simulink model "Fusion_Frame_Model_Architecture"  (R2018a)
settings: Solver=FixedStepAuto  StartTime=0.0  StopTime=SimulationTime  FixedStep=SamplingTime  RelTol=1e-3
undefined symbols (not defined in the file or in its folder): ACTIVATE_CAM, ACTIVATE_RAD, CAM1_detTimeStamp, CAM1_MeasNoise, CAM1_objClassID, CAM1_PX, CAM1_PY, CAM1_VX, CAM1_VY, CAM2_detTimeStamp, CAM2_MeasNoise, CAM2_objClassID, CAM2_PX, CAM2_PY, CAM2_VX, CAM2_VY, CAM3_detTimeStamp, CAM3_MeasNoise, CAM3_objClassID, CAM3_PX, CAM3_PY, CAM3_VX, CAM3_VY, CAM4_detTimeStamp, CAM4_MeasNoise, CAM4_objClassID, CAM4_PX, CAM4_PY, CAM4_VX, CAM4_VY, CAM5_detTimeStamp, CAM5_MeasNoise, CAM5_objClassID, CAM5_PX, CAM5_PY, CAM5_VX, CAM5_VY, CAM6_detTimeStamp, CAM6_MeasNoise, CAM6_objClassID, CAM6_PX, CAM6_PY, CAM6_VX, CAM6_VY, CAM7_detTimeStamp, CAM7_MeasNoise, CAM7_objClassID, CAM7_PX, CAM7_PY, CAM7_VX, CAM7_VY, CAM8_detTimeStamp, CAM8_MeasNoise, CAM8_objClassID, CAM8_PX, CAM8_PY, CAM8_VX, CAM8_VY, CAM_nMeas, CAM_TYPE ... (+181)
libraries: simulink_extras x4
(part 3 of 11)

== system Fusion_Frame_Model_Architecture/SENSOR_MEASUREMENTS/RADAR_CAMERA_EGO_SENSOR_INTERFACE/CameraSensors/Camera7 ==
  timeIdx : Inport
  nObjCamera : Inport  Port=2
  SensorMeas : Inport  Port=3
  ExtractMeasParam1 : Subsystem
  For Iterator : ForIterator  ResetStates=reset  IterationSource=external  IterationVariableDataType=int16
  IsValid2 : Subsystem
  Selector : Selector  InputPortWidth=nCameras  IndexOptions=Starting index (dialog)  Indices=7  OutputSizes=1
  Subsystem1 : Subsystem
  C7 : Outport
  wires:
  ExtractMeasParam1/1(PX) -> IsValid2/2(px), [px]
  ExtractMeasParam1/7(measCaptureTime) -> Subsystem1/9(TIME_STAMP)
  IsValid2/1(ID) -> Subsystem1/6(id)
  [vy] -> Subsystem1/5(vy)  "vy"
  ExtractMeasParam1/6(NOISE_COV) -> Subsystem1/8(NOISE_COV)
  [vx] -> Subsystem1/4(vx)  "vx"
  SensorMeas/1 -> Subsystem1/1(SensorData)
  nObjCamera/1 -> Selector/1
  [py] -> Subsystem1/3(py)  "py"
  For Iterator/1 -> [index]
  [index] -> Subsystem1/10(iter), IsValid2/1(idx), ExtractMeasParam1/1(idx)
  ExtractMeasParam1/4(VY) -> IsValid2/5(vy), [vy]
  [px] -> Subsystem1/2(px)  "px"
  Selector/1 -> For Iterator/1
  ExtractMeasParam1/2(PY) -> IsValid2/3(py), [py]
  Subsystem1/1(C7) -> C7/1
  ExtractMeasParam1/5(OBJ_TYPE) -> Subsystem1/7(OBJ_TYPE)
  timeIdx/1 -> ExtractMeasParam1/2(time)
  ExtractMeasParam1/3(VX) -> IsValid2/4(vx), [vx]

== system Fusion_Frame_Model_Architecture/SENSOR_MEASUREMENTS/RADAR_CAMERA_EGO_SENSOR_INTERFACE/CameraSensors/Camera8 ==
  timeIdx : Inport
  nObjCamera : Inport  Port=2
  SensorMeas : Inport  Port=3
  ExtractMeasParam1 : Subsystem
  For Iterator : ForIterator  ResetStates=reset  IterationSource=external  IterationVariableDataType=int16
  IsValid2 : Subsystem
  Selector : Selector  InputPortWidth=nCameras  IndexOptions=Starting index (dialog)  Indices=8  OutputSizes=1
  Subsystem1 : Subsystem
  C8 : Outport
  wires:
  ExtractMeasParam1/1(PX) -> IsValid2/2(px), [px]
  ExtractMeasParam1/7(measCaptureTime) -> Subsystem1/9(TIME_STAMP)
  IsValid2/1(ID) -> Subsystem1/6(id)
  [vy] -> Subsystem1/5(vy)  "vy"
  ExtractMeasParam1/6(NOISE_COV) -> Subsystem1/8(NOISE_COV)
  [vx] -> Subsystem1/4(vx)  "vx"
  SensorMeas/1 -> Subsystem1/1(SensorData)
  nObjCamera/1 -> Selector/1
  [py] -> Subsystem1/3(py)  "py"
  For Iterator/1 -> [index]
  [index] -> Subsystem1/10(iter), IsValid2/1(idx), ExtractMeasParam1/1(idx)
  ExtractMeasParam1/4(VY) -> IsValid2/5(vy), [vy]
  [px] -> Subsystem1/2(px)  "px"
  Selector/1 -> For Iterator/1
  ExtractMeasParam1/2(PY) -> IsValid2/3(py), [py]
  Subsystem1/1(C8) -> C8/1
  ExtractMeasParam1/5(OBJ_TYPE) -> Subsystem1/7(OBJ_TYPE)
  timeIdx/1 -> ExtractMeasParam1/2(time)
  ExtractMeasParam1/3(VX) -> IsValid2/4(vx), [vx]

== system Fusion_Frame_Model_Architecture/SENSOR_MEASUREMENTS/RADAR_CAMERA_EGO_SENSOR_INTERFACE/EgoSensors/ExtractMeasParam ==
  timeIdx : Inport
  Constant : Constant  Value=EGO_PX
  Constant1 : Constant  Value=EGO_PY
  Constant2 : Constant  Value=EGO_VX
  Constant3 : Constant  Value=EGO_VY
  Constant4 : Constant  Value=EGO_YAW
  Constant5 : Constant  Value=EGO_YAWRATE
  Constant6 : Constant  Value=EGO_TimeStamp
  Constant7 : Constant  Value=EGO_IgnitionStatus
  EGO_PX : Selector  NumberOfDimensions=2  InputPortWidth=portSize  IndexOptions=Select all,Index vector (port)  Indices=[1 3],1  OutputSizes=1,1
  EGO_PY : Selector  NumberOfDimensions=2  InputPortWidth=portSize  IndexOptions=Select all,Index vector (port)  Indices=[1 3],1  OutputSizes=1,1
  EGO_VX : Selector  NumberOfDimensions=2  InputPortWidth=portSize  IndexOptions=Select all,Index vector (port)  Indices=[1 3],1  OutputSizes=1,1
  EGO_VY : Selector  NumberOfDimensions=2  InputPortWidth=portSize  IndexOptions=Select all,Index vector (port)  Indices=[1 3],1  OutputSizes=1,1
  EGO_YAW : Selector  NumberOfDimensions=2  InputPortWidth=portSize  IndexOptions=Select all,Index vector (port)  Indices=[1 3],1  OutputSizes=1,1
  EGO_YAWRATE : Selector  NumberOfDimensions=2  InputPortWidth=portSize  IndexOptions=Select all,Index vector (port)  Indices=[1 3],1  OutputSizes=1,1
  TIME_STAMP : Selector  NumberOfDimensions=2  InputPortWidth=portSize  IndexOptions=Select all,Index vector (port)  Indices=[1 3],1  OutputSizes=1,1
  TIME_STAMP1 : Selector  NumberOfDimensions=2  InputPortWidth=portSize  IndexOptions=Select all,Index vector (port)  Indices=[1 3],1  OutputSizes=1,1
  EgoTimeStamp : Outport
  EgoPx : Outport  Port=2
  EgoPy : Outport  Port=3
  EgoVx : Outport  Port=4
  EgoVy : Outport  Port=5
  EgoYaw : Outport  Port=6
  EgoYawRate : Outport  Port=7
  EgoIgnitionStatus : Outport  Port=8
  wires:
  Constant3/1 -> EGO_VY/1
  Constant2/1 -> EGO_VX/1
  Constant/1 -> EGO_PX/1
  Constant1/1 -> EGO_PY/1
  EGO_VX/1 -> EgoVx/1
  EGO_PX/1 -> EgoPx/1
  timeIdx/1 -> EGO_PX/2, EGO_PY/2, EGO_VX/2, EGO_VY/2, EGO_YAW/2, EGO_YAWRATE/2, TIME_STAMP1/2, TIME_STAMP/2
  Constant4/1 -> EGO_YAW/1
  EGO_YAW/1 -> EgoYaw/1
  Constant6/1 -> TIME_STAMP/1
  TIME_STAMP/1 -> EgoTimeStamp/1
  EGO_YAWRATE/1 -> EgoYawRate/1
  Constant5/1 -> EGO_YAWRATE/1
  EGO_PY/1 -> EgoPy/1
  EGO_VY/1 -> EgoVy/1
  Constant7/1 -> TIME_STAMP1/1
  TIME_STAMP1/1 -> EgoIgnitionStatus/1

== system Fusion_Frame_Model_Architecture/SENSOR_MEASUREMENTS/RADAR_CAMERA_EGO_SENSOR_INTERFACE/RadarSensors/Radar1 ==
  timeIdx : Inport
  nObjRadar : Inport  Port=2
  SensorMeas : Inport  Port=3
  CHECK_IF_DATA_VALID : Subsystem
  GET_DATA : Subsystem
  LOOP_OVER_RADARS : ForIterator  ResetStates=reset  IterationSource=external  IterationVariableDataType=int16
  SET_DATA : Subsystem
  Selector : Selector  InputPortWidth=nRadars  IndexOptions=Starting index (dialog)  Indices=1  OutputSizes=1
  R1 : Outport
  wires:
  nObjRadar/1 -> Selector/1
  LOOP_OVER_RADARS/1 -> [index]
  [index] -> CHECK_IF_DATA_VALID/1(idx), GET_DATA/1(idx), SET_DATA/10(iter)
  timeIdx/1 -> GET_DATA/2(time)
  GET_DATA/1(PX) -> CHECK_IF_DATA_VALID/2(px), [px]
  GET_DATA/2(PY) -> CHECK_IF_DATA_VALID/3(py), [py]
  GET_DATA/3(VX) -> CHECK_IF_DATA_VALID/4(vx), [vx]
  GET_DATA/4(VY) -> CHECK_IF_DATA_VALID/5(vy), [vy]
  SensorMeas/1 -> SET_DATA/1(SensorData)
  [px] -> SET_DATA/2(px)  "px"
  [py] -> SET_DATA/3(py)  "py"
  [vx] -> SET_DATA/4(vx)  "vx"
  [vy] -> SET_DATA/5(vy)  "vy"
  SET_DATA/1(R1) -> R1/1
  CHECK_IF_DATA_VALID/1(ID) -> SET_DATA/6(id)
  Selector/1 -> LOOP_OVER_RADARS/1
  GET_DATA/5(SNR) -> SET_DATA/7(SNR)
  GET_DATA/6(NOISE_COV) -> SET_DATA/8(NOISE_COV)
  GET_DATA/7(measCaptureTime) -> SET_DATA/9(TIME_STAMP)

== system Fusion_Frame_Model_Architecture/SENSOR_MEASUREMENTS/RADAR_CAMERA_EGO_SENSOR_INTERFACE/RadarSensors/Radar2 ==
  timeIdx : Inport
  nObjRadar : Inport  Port=2
  SensorMeas : Inport  Port=3
  ExtractMeasParam : Subsystem
  For Iterator : ForIterator  ResetStates=reset  IterationSource=external  IterationVariableDataType=int16
  IsValid1 : Subsystem
  Selector : Selector  InputPortWidth=nRadars  IndexOptions=Starting index (dialog)  Indices=2  OutputSizes=1
  Subsystem : Subsystem
  R2 : Outport
  wires:
  [vx] -> Subsystem/4(vx)  "vx"
  Subsystem/1(R2) -> R2/1
  ExtractMeasParam/1(PX) -> IsValid1/2(px), [px]
  IsValid1/1(ID) -> Subsystem/6(id)
  [py] -> Subsystem/3(py)  "py"
  ExtractMeasParam/3(VX) -> IsValid1/4(vx), [vx]
  ExtractMeasParam/6(NOISE_COV) -> Subsystem/8(NOISE_COV)
  ExtractMeasParam/4(VY) -> IsValid1/5(vy), [vy]
  [px] -> Subsystem/2(px)  "px"
  nObjRadar/1 -> Selector/1
  SensorMeas/1 -> Subsystem/1(SensorData)
  timeIdx/1 -> ExtractMeasParam/2(time)
  [index] -> IsValid1/1(idx), ExtractMeasParam/1(idx), Subsystem/10(iter)
  [vy] -> Subsystem/5(vy)  "vy"
  ExtractMeasParam/2(PY) -> IsValid1/3(py), [py]
  For Iterator/1 -> [index]
  ExtractMeasParam/5(SNR) -> Subsystem/7(SNR)
  ExtractMeasParam/7(measCaptureTime) -> Subsystem/9(TIME_STAMP)
  Selector/1 -> For Iterator/1

== system Fusion_Frame_Model_Architecture/SENSOR_MEASUREMENTS/RADAR_CAMERA_EGO_SENSOR_INTERFACE/RadarSensors/Radar3 ==
  timeIdx : Inport
  nObjRadar : Inport  Port=2
  SensorMeas : Inport  Port=3
  ExtractMeasParam : Subsystem
  For Iterator : ForIterator  ResetStates=reset  IterationSource=external  IterationVariableDataType=int16
  IsValid1 : Subsystem
  Selector : Selector  InputPortWidth=nRadars  IndexOptions=Starting index (dialog)  Indices=3  OutputSizes=1
  Subsystem : Subsystem
  R3 : Outport
  wires:
  [vx] -> Subsystem/4(vx)  "vx"
  Subsystem/1(R3) -> R3/1
  ExtractMeasParam/1(PX) -> IsValid1/2(px), [px]
  IsValid1/1(ID) -> Subsystem/6(id)
  [py] -> Subsystem/3(py)  "py"
  ExtractMeasParam/3(VX) -> IsValid1/4(vx), [vx]
  ExtractMeasParam/6(NOISE_COV) -> Subsystem/8(NOISE_COV)
  ExtractMeasParam/4(VY) -> IsValid1/5(vy), [vy]
  [px] -> Subsystem/2(px)  "px"
  nObjRadar/1 -> Selector/1
  SensorMeas/1 -> Subsystem/1(SensorData)
  timeIdx/1 -> ExtractMeasParam/2(time)
  [index] -> IsValid1/1(idx), ExtractMeasParam/1(idx), Subsystem/10(iter)
  [vy] -> Subsystem/5(vy)  "vy"
  ExtractMeasParam/2(PY) -> IsValid1/3(py), [py]
  For Iterator/1 -> [index]
  ExtractMeasParam/5(SNR) -> Subsystem/7(SNR)
  ExtractMeasParam/7(measCaptureTime) -> Subsystem/9(TIME_STAMP)
  Selector/1 -> For Iterator/1

== system Fusion_Frame_Model_Architecture/SENSOR_MEASUREMENTS/RADAR_CAMERA_EGO_SENSOR_INTERFACE/RadarSensors/Radar4 ==
  timeIdx : Inport
  nObjRadar : Inport  Port=2
  SensorMeas : Inport  Port=3
  ExtractMeasParam : Subsystem
  For Iterator : ForIterator  ResetStates=reset  IterationSource=external  IterationVariableDataType=int16
  IsValid1 : Subsystem
  Selector : Selector  InputPortWidth=nRadars  IndexOptions=Starting index (dialog)  Indices=4  OutputSizes=1
  Subsystem : Subsystem
  R4 : Outport
  wires:
  ExtractMeasParam/2(PY) -> IsValid1/3(py), [py]
  [vy] -> Subsystem/5(vy)  "vy"
  [index] -> IsValid1/1(idx), ExtractMeasParam/1(idx), Subsystem/10(iter)
  SensorMeas/1 -> Subsystem/1(SensorData)
  ExtractMeasParam/6(NOISE_COV) -> Subsystem/8(NOISE_COV)
  ExtractMeasParam/4(VY) -> IsValid1/5(vy), [vy]
  ExtractMeasParam/3(VX) -> IsValid1/4(vx), [vx]
  timeIdx/1 -> ExtractMeasParam/2(time)
  IsValid1/1(ID) -> Subsystem/6(id)
  ExtractMeasParam/1(PX) -> IsValid1/2(px), [px]
  [vx] -> Subsystem/4(vx)  "vx"
  Selector/1 -> For Iterator/1
  nObjRadar/1 -> Selector/1
  Subsystem/1(R4) -> R4/1
  ExtractMeasParam/7(measCaptureTime) -> Subsystem/9(TIME_STAMP)
  [px] -> Subsystem/2(px)  "px"
  ExtractMeasParam/5(SNR) -> Subsystem/7(SNR)
  [py] -> Subsystem/3(py)  "py"
  For Iterator/1 -> [index]

== system Fusion_Frame_Model_Architecture/SENSOR_MEASUREMENTS/RADAR_CAMERA_EGO_SENSOR_INTERFACE/RadarSensors/Radar5 ==
  timeIdx : Inport
  nObjRadar : Inport  Port=2
  SensorMeas : Inport  Port=3
  ExtractMeasParam : Subsystem
  For Iterator : ForIterator  ResetStates=reset  IterationSource=external  IterationVariableDataType=int16
  IsValid1 : Subsystem
  Selector : Selector  InputPortWidth=nRadars  IndexOptions=Starting index (dialog)  Indices=5  OutputSizes=1
  Subsystem : Subsystem
  R5 : Outport
  wires:
  ExtractMeasParam/2(PY) -> IsValid1/3(py), [py]
  [vy] -> Subsystem/5(vy)  "vy"
  [index] -> IsValid1/1(idx), ExtractMeasParam/1(idx), Subsystem/10(iter)
  SensorMeas/1 -> Subsystem/1(SensorData)
  ExtractMeasParam/6(NOISE_COV) -> Subsystem/8(NOISE_COV)
  ExtractMeasParam/4(VY) -> IsValid1/5(vy), [vy]
  ExtractMeasParam/3(VX) -> IsValid1/4(vx), [vx]
  timeIdx/1 -> ExtractMeasParam/2(time)
  IsValid1/1(ID) -> Subsystem/6(id)
  ExtractMeasParam/1(PX) -> IsValid1/2(px), [px]
  [vx] -> Subsystem/4(vx)  "vx"
  Selector/1 -> For Iterator/1
  nObjRadar/1 -> Selector/1
  Subsystem/1(R5) -> R5/1
  ExtractMeasParam/7(measCaptureTime) -> Subsystem/9(TIME_STAMP)
  [px] -> Subsystem/2(px)  "px"
  ExtractMeasParam/5(SNR) -> Subsystem/7(SNR)
  [py] -> Subsystem/3(py)  "py"
  For Iterator/1 -> [index]

== system Fusion_Frame_Model_Architecture/SENSOR_MEASUREMENTS/RADAR_CAMERA_EGO_SENSOR_INTERFACE/RadarSensors/Radar6 ==
  timeIdx : Inport
  nObjRadar : Inport  Port=2
  SensorMeas : Inport  Port=3
  ExtractMeasParam : Subsystem
  For Iterator : ForIterator  ResetStates=reset  IterationSource=external  IterationVariableDataType=int16
  IsValid1 : Subsystem
  Selector : Selector  InputPortWidth=nRadars  IndexOptions=Starting index (dialog)  Indices=6  OutputSizes=1
  Subsystem : Subsystem
  R6 : Outport
  wires:
  ExtractMeasParam/2(PY) -> IsValid1/3(py), [py]
  [vy] -> Subsystem/5(vy)  "vy"
  [index] -> IsValid1/1(idx), ExtractMeasParam/1(idx), Subsystem/10(iter)
  SensorMeas/1 -> Subsystem/1(SensorData)
  ExtractMeasParam/6(NOISE_COV) -> Subsystem/8(NOISE_COV)
  ExtractMeasParam/4(VY) -> IsValid1/5(vy), [vy]
  ExtractMeasParam/3(VX) -> IsValid1/4(vx), [vx]
  timeIdx/1 -> ExtractMeasParam/2(time)
  IsValid1/1(ID) -> Subsystem/6(id)
  ExtractMeasParam/1(PX) -> IsValid1/2(px), [px]
  [vx] -> Subsystem/4(vx)  "vx"
  Selector/1 -> For Iterator/1
  nObjRadar/1 -> Selector/1
  Subsystem/1(R6) -> R6/1
  ExtractMeasParam/7(measCaptureTime) -> Subsystem/9(TIME_STAMP)
  [px] -> Subsystem/2(px)  "px"
  ExtractMeasParam/5(SNR) -> Subsystem/7(SNR)
  [py] -> Subsystem/3(py)  "py"
  For Iterator/1 -> [index]

== system Fusion_Frame_Model_Architecture/SENSOR_MEASUREMENTS/RADAR_CAMERA_EGO_SENSOR_INTERFACE/RoadSensors/Camera1 ==
  timeIdx : Inport
  nLines : Inport  Port=2
  CameraLineCoeff : Inport  Port=3
  CHECK_IF_DATA_IS_VALID : Subsystem
  GET_DATA : Subsystem
  LOOP_OVER_CAMERAS : ForIterator  ResetStates=reset  IterationSource=external  IterationVariableDataType=int16
  SET_DATA : Subsystem
  Selector : Selector  InputPortWidth=nCameras  IndexOptions=Index vector (dialog)  Indices=1  OutputSizes=1
  C1 : Outport
  wires:
  nLines/1 -> Selector/1
  LOOP_OVER_CAMERAS/1 -> [index]
  GET_DATA/5(lateralOffset) -> SET_DATA/7(lateralOffset)
  [curv] -> SET_DATA/2(curv)
  GET_DATA/9(measCaptureTime) -> SET_DATA/11(TIME_STAMP)
  SET_DATA/1(C1) -> C1/1
  [curvLen] -> SET_DATA/4(curvLen)
  GET_DATA/1(curvature) -> CHECK_IF_DATA_IS_VALID/2(curvature), [curv]
  Selector/1 -> LOOP_OVER_CAMERAS/1
  GET_DATA/3(curvLength) -> CHECK_IF_DATA_IS_VALID/4(curvLength), [curvLen]
  timeIdx/1 -> GET_DATA/2(time)
  CHECK_IF_DATA_IS_VALID/1(validID) -> SET_DATA/6(ValidID)
  CameraLineCoeff/1 -> SET_DATA/1(CameraLineCoeff)
  GET_DATA/6(xmin) -> SET_DATA/8(xmin)
  [alpha] -> SET_DATA/5(alpha)
  [curvRate] -> SET_DATA/3(curvRate)
  GET_DATA/4(headingAngle) -> CHECK_IF_DATA_IS_VALID/5(HeadingAngle), [alpha]
  GET_DATA/2(curvRate) -> CHECK_IF_DATA_IS_VALID/3(curvatureRate), [curvRate]
  [index] -> CHECK_IF_DATA_IS_VALID/1(LineID), SET_DATA/12(iter), GET_DATA/1(idx)
  GET_DATA/7(xmax) -> SET_DATA/9(xmax)
  GET_DATA/8(lineMarkWidth) -> SET_DATA/10(lineWidth)

== system Fusion_Frame_Model_Architecture/SENSOR_MEASUREMENTS/RADAR_CAMERA_EGO_SENSOR_INTERFACE/RoadSensors/Camera2 ==
  timeIdx : Inport
  nLines : Inport  Port=2
  CameraLineCoeff : Inport  Port=3
  ExtractMeasParam1 : Subsystem
  For Iterator : ForIterator  ResetStates=reset  IterationSource=external  IterationVariableDataType=int16
  IsValid2 : Subsystem
  Selector : Selector  InputPortWidth=nCameras  IndexOptions=Index vector (dialog)  Indices=2  OutputSizes=1
  Subsystem1 : Subsystem
  C1 : Outport
  wires:
  ExtractMeasParam1/7(xmax) -> Subsystem1/9(xmax)
  ExtractMeasParam1/8(lineMarkWidth) -> Subsystem1/10(lineWidth)
  [index] -> IsValid2/1(LineID), Subsystem1/12(iter), ExtractMeasParam1/1(idx)
  timeIdx/1 -> ExtractMeasParam1/2(time)
  ExtractMeasParam1/2(curvRate) -> IsValid2/3(curvatureRate), [curvRate]
  [curvRate] -> Subsystem1/3(curvRate)
  [curv] -> Subsystem1/2(curv)
  ExtractMeasParam1/3(curvLength) -> IsValid2/4(curvLength), [curvLen]
  ExtractMeasParam1/1(curvature) -> IsValid2/2(curvature), [curv]
  Subsystem1/1(C1) -> C1/1
  [curvLen] -> Subsystem1/4(curvLen)
  For Iterator/1 -> [index]
  ExtractMeasParam1/4(headingAngle) -> IsValid2/5(HeadingAngle), [alpha]
  ExtractMeasParam1/5(lateralOffset) -> Subsystem1/7(lateralOffset)
  Selector/1 -> For Iterator/1
  IsValid2/1(validID) -> Subsystem1/6(ValidID)
  ExtractMeasParam1/6(xmin) -> Subsystem1/8(xmin)
  CameraLineCoeff/1 -> Subsystem1/1(CameraLineCoeff)
  nLines/1 -> Selector/1
  ExtractMeasParam1/9(measCaptureTime) -> Subsystem1/11(TIME_STAMP)
  [alpha] -> Subsystem1/5(alpha)

== system Fusion_Frame_Model_Architecture/SENSOR_MEASUREMENTS/RADAR_CAMERA_EGO_SENSOR_INTERFACE/RoadSensors/Camera3 ==
  timeIdx : Inport
  nLines : Inport  Port=2
  CameraLineCoeff : Inport  Port=3
  ExtractMeasParam1 : Subsystem
  For Iterator : ForIterator  ResetStates=reset  IterationSource=external  IterationVariableDataType=int16
  IsValid2 : Subsystem
  Selector : Selector  InputPortWidth=nCameras  IndexOptions=Index vector (dialog)  Indices=3  OutputSizes=1
  Subsystem1 : Subsystem
  C1 : Outport
  wires:
  ExtractMeasParam1/7(xmax) -> Subsystem1/9(xmax)
  ExtractMeasParam1/8(lineMarkWidth) -> Subsystem1/10(lineWidth)
  [index] -> IsValid2/1(LineID), Subsystem1/12(iter), ExtractMeasParam1/1(idx)
  timeIdx/1 -> ExtractMeasParam1/2(time)
  ExtractMeasParam1/2(curvRate) -> IsValid2/3(curvatureRate), [curvRate]
  [curvRate] -> Subsystem1/3(curvRate)
  [curv] -> Subsystem1/2(curv)
  ExtractMeasParam1/3(curvLength) -> IsValid2/4(curvLength), [curvLen]
  ExtractMeasParam1/1(curvature) -> IsValid2/2(curvature), [curv]
  Subsystem1/1(C1) -> C1/1
  [curvLen] -> Subsystem1/4(curvLen)
  For Iterator/1 -> [index]
  ExtractMeasParam1/4(headingAngle) -> IsValid2/5(HeadingAngle), [alpha]
  ExtractMeasParam1/5(lateralOffset) -> Subsystem1/7(lateralOffset)
  Selector/1 -> For Iterator/1
  IsValid2/1(validID) -> Subsystem1/6(ValidID)
  ExtractMeasParam1/6(xmin) -> Subsystem1/8(xmin)
  CameraLineCoeff/1 -> Subsystem1/1(CameraLineCoeff)
  nLines/1 -> Selector/1
  ExtractMeasParam1/9(measCaptureTime) -> Subsystem1/11(TIME_STAMP)
  [alpha] -> Subsystem1/5(alpha)

== system Fusion_Frame_Model_Architecture/SENSOR_MEASUREMENTS/RADAR_CAMERA_EGO_SENSOR_INTERFACE/RoadSensors/Camera4 ==
  timeIdx : Inport
  nLines : Inport  Port=2
  CameraLineCoeff : Inport  Port=3
  ExtractMeasParam1 : Subsystem
  For Iterator : ForIterator  ResetStates=reset  IterationSource=external  IterationVariableDataType=int16
  IsValid2 : Subsystem
  Selector : Selector  InputPortWidth=nCameras  IndexOptions=Index vector (dialog)  Indices=4  OutputSizes=1
  Subsystem1 : Subsystem
  C1 : Outport
  wires:
  ExtractMeasParam1/7(xmax) -> Subsystem1/9(xmax)
  ExtractMeasParam1/8(lineMarkWidth) -> Subsystem1/10(lineWidth)
  [index] -> IsValid2/1(LineID), Subsystem1/12(iter), ExtractMeasParam1/1(idx)
  timeIdx/1 -> ExtractMeasParam1/2(time)
  ExtractMeasParam1/2(curvRate) -> IsValid2/3(curvatureRate), [curvRate]
  [curvRate] -> Subsystem1/3(curvRate)
  [curv] -> Subsystem1/2(curv)
  ExtractMeasParam1/3(curvLength) -> IsValid2/4(curvLength), [curvLen]
  ExtractMeasParam1/1(curvature) -> IsValid2/2(curvature), [curv]
  Subsystem1/1(C1) -> C1/1
  [curvLen] -> Subsystem1/4(curvLen)
  For Iterator/1 -> [index]
  ExtractMeasParam1/4(headingAngle) -> IsValid2/5(HeadingAngle), [alpha]
  ExtractMeasParam1/5(lateralOffset) -> Subsystem1/7(lateralOffset)
  Selector/1 -> For Iterator/1
  IsValid2/1(validID) -> Subsystem1/6(ValidID)
  ExtractMeasParam1/6(xmin) -> Subsystem1/8(xmin)
  CameraLineCoeff/1 -> Subsystem1/1(CameraLineCoeff)
  nLines/1 -> Selector/1
  ExtractMeasParam1/9(measCaptureTime) -> Subsystem1/11(TIME_STAMP)
  [alpha] -> Subsystem1/5(alpha)

== system Fusion_Frame_Model_Architecture/SENSOR_MEASUREMENTS/RADAR_CAMERA_EGO_SENSOR_INTERFACE/RoadSensors/Camera5 ==
  timeIdx : Inport
  nLines : Inport  Port=2
  CameraLineCoeff : Inport  Port=3
  ExtractMeasParam1 : Subsystem
  For Iterator : ForIterator  ResetStates=reset  IterationSource=external  IterationVariableDataType=int16
  IsValid2 : Subsystem
  Selector : Selector  InputPortWidth=nCameras  IndexOptions=Index vector (dialog)  Indices=5  OutputSizes=1
  Subsystem1 : Subsystem
  C1 : Outport
  wires:
  ExtractMeasParam1/7(xmax) -> Subsystem1/9(xmax)
  ExtractMeasParam1/8(lineMarkWidth) -> Subsystem1/10(lineWidth)
  [index] -> IsValid2/1(LineID), Subsystem1/12(iter), ExtractMeasParam1/1(idx)
  timeIdx/1 -> ExtractMeasParam1/2(time)
  ExtractMeasParam1/2(curvRate) -> IsValid2/3(curvatureRate), [curvRate]
  [curvRate] -> Subsystem1/3(curvRate)
  [curv] -> Subsystem1/2(curv)
  ExtractMeasParam1/3(curvLength) -> IsValid2/4(curvLength), [curvLen]
  ExtractMeasParam1/1(curvature) -> IsValid2/2(curvature), [curv]
  Subsystem1/1(C1) -> C1/1
  [curvLen] -> Subsystem1/4(curvLen)
  For Iterator/1 -> [index]
  ExtractMeasParam1/4(headingAngle) -> IsValid2/5(HeadingAngle), [alpha]
  ExtractMeasParam1/5(lateralOffset) -> Subsystem1/7(lateralOffset)
  Selector/1 -> For Iterator/1
  IsValid2/1(validID) -> Subsystem1/6(ValidID)
  ExtractMeasParam1/6(xmin) -> Subsystem1/8(xmin)
  CameraLineCoeff/1 -> Subsystem1/1(CameraLineCoeff)
  nLines/1 -> Selector/1
  ExtractMeasParam1/9(measCaptureTime) -> Subsystem1/11(TIME_STAMP)
  [alpha] -> Subsystem1/5(alpha)

== system Fusion_Frame_Model_Architecture/SENSOR_MEASUREMENTS/RADAR_CAMERA_EGO_SENSOR_INTERFACE/RoadSensors/Camera6 ==
  timeIdx : Inport
  nLines : Inport  Port=2
  CameraLineCoeff : Inport  Port=3
  ExtractMeasParam1 : Subsystem
  For Iterator : ForIterator  ResetStates=reset  IterationSource=external  IterationVariableDataType=int16
  IsValid2 : Subsystem
  Selector : Selector  InputPortWidth=nCameras  IndexOptions=Index vector (dialog)  Indices=6  OutputSizes=1
  Subsystem1 : Subsystem
  C1 : Outport
  wires:
  ExtractMeasParam1/7(xmax) -> Subsystem1/9(xmax)
  ExtractMeasParam1/8(lineMarkWidth) -> Subsystem1/10(lineWidth)
  [index] -> IsValid2/1(LineID), Subsystem1/12(iter), ExtractMeasParam1/1(idx)
  timeIdx/1 -> ExtractMeasParam1/2(time)
  ExtractMeasParam1/2(curvRate) -> IsValid2/3(curvatureRate), [curvRate]
  [curvRate] -> Subsystem1/3(curvRate)
  [curv] -> Subsystem1/2(curv)
  ExtractMeasParam1/3(curvLength) -> IsValid2/4(curvLength), [curvLen]
  ExtractMeasParam1/1(curvature) -> IsValid2/2(curvature), [curv]
  Subsystem1/1(C1) -> C1/1
  [curvLen] -> Subsystem1/4(curvLen)
  For Iterator/1 -> [index]
  ExtractMeasParam1/4(headingAngle) -> IsValid2/5(HeadingAngle), [alpha]
  ExtractMeasParam1/5(lateralOffset) -> Subsystem1/7(lateralOffset)
  Selector/1 -> For Iterator/1
  IsValid2/1(validID) -> Subsystem1/6(ValidID)
  ExtractMeasParam1/6(xmin) -> Subsystem1/8(xmin)
  CameraLineCoeff/1 -> Subsystem1/1(CameraLineCoeff)
  nLines/1 -> Selector/1
  ExtractMeasParam1/9(measCaptureTime) -> Subsystem1/11(TIME_STAMP)
  [alpha] -> Subsystem1/5(alpha)

== system Fusion_Frame_Model_Architecture/SENSOR_MEASUREMENTS/RADAR_CAMERA_EGO_SENSOR_INTERFACE/RoadSensors/Camera7 ==
  timeIdx : Inport
  nLines : Inport  Port=2
  CameraLineCoeff : Inport  Port=3
  ExtractMeasParam1 : Subsystem
  For Iterator : ForIterator  ResetStates=reset  IterationSource=external  IterationVariableDataType=int16
  IsValid2 : Subsystem
  Selector : Selector  InputPortWidth=nCameras  IndexOptions=Index vector (dialog)  Indices=7  OutputSizes=1
  Subsystem1 : Subsystem
  C1 : Outport
  wires:
  ExtractMeasParam1/7(xmax) -> Subsystem1/9(xmax)
  ExtractMeasParam1/8(lineMarkWidth) -> Subsystem1/10(lineWidth)
  [index] -> IsValid2/1(LineID), Subsystem1/12(iter), ExtractMeasParam1/1(idx)
  timeIdx/1 -> ExtractMeasParam1/2(time)
  ExtractMeasParam1/2(curvRate) -> IsValid2/3(curvatureRate), [curvRate]
  [curvRate] -> Subsystem1/3(curvRate)
  [curv] -> Subsystem1/2(curv)
  ExtractMeasParam1/3(curvLength) -> IsValid2/4(curvLength), [curvLen]
  ExtractMeasParam1/1(curvature) -> IsValid2/2(curvature), [curv]
  Subsystem1/1(C1) -> C1/1
  [curvLen] -> Subsystem1/4(curvLen)
  For Iterator/1 -> [index]
  ExtractMeasParam1/4(headingAngle) -> IsValid2/5(HeadingAngle), [alpha]
  ExtractMeasParam1/5(lateralOffset) -> Subsystem1/7(lateralOffset)
  Selector/1 -> For Iterator/1
  IsValid2/1(validID) -> Subsystem1/6(ValidID)
  ExtractMeasParam1/6(xmin) -> Subsystem1/8(xmin)
  CameraLineCoeff/1 -> Subsystem1/1(CameraLineCoeff)
  nLines/1 -> Selector/1
  ExtractMeasParam1/9(measCaptureTime) -> Subsystem1/11(TIME_STAMP)
  [alpha] -> Subsystem1/5(alpha)

== system Fusion_Frame_Model_Architecture/SENSOR_MEASUREMENTS/RADAR_CAMERA_EGO_SENSOR_INTERFACE/RoadSensors/Camera8 ==
  timeIdx : Inport
  nLines : Inport  Port=2
  CameraLineCoeff : Inport  Port=3
  ExtractMeasParam1 : Subsystem
  For Iterator : ForIterator  ResetStates=reset  IterationSource=external  IterationVariableDataType=int16
  IsValid2 : Subsystem
  Selector : Selector  InputPortWidth=nCameras  IndexOptions=Index vector (dialog)  Indices=8  OutputSizes=1
  Subsystem1 : Subsystem
  C1 : Outport
  wires:
  ExtractMeasParam1/7(xmax) -> Subsystem1/9(xmax)
  ExtractMeasParam1/8(lineMarkWidth) -> Subsystem1/10(lineWidth)
  [index] -> IsValid2/1(LineID), Subsystem1/12(iter), ExtractMeasParam1/1(idx)
  timeIdx/1 -> ExtractMeasParam1/2(time)
  ExtractMeasParam1/2(curvRate) -> IsValid2/3(curvatureRate), [curvRate]
  [curvRate] -> Subsystem1/3(curvRate)
  [curv] -> Subsystem1/2(curv)
  ExtractMeasParam1/3(curvLength) -> IsValid2/4(curvLength), [curvLen]
  ExtractMeasParam1/1(curvature) -> IsValid2/2(curvature), [curv]
  Subsystem1/1(C1) -> C1/1
  [curvLen] -> Subsystem1/4(curvLen)
  For Iterator/1 -> [index]
  ExtractMeasParam1/4(headingAngle) -> IsValid2/5(HeadingAngle), [alpha]
  ExtractMeasParam1/5(lateralOffset) -> Subsystem1/7(lateralOffset)
  Selector/1 -> For Iterator/1
  IsValid2/1(validID) -> Subsystem1/6(ValidID)
  ExtractMeasParam1/6(xmin) -> Subsystem1/8(xmin)
  CameraLineCoeff/1 -> Subsystem1/1(CameraLineCoeff)
  nLines/1 -> Selector/1
  ExtractMeasParam1/9(measCaptureTime) -> Subsystem1/11(TIME_STAMP)
  [alpha] -> Subsystem1/5(alpha)

== system Fusion_Frame_Model_Architecture/SENSOR_FUSION_SYSTEM/OBJECT_TRACKER_SENSOR_FUSION/CAMERA_HOMOGENEOUS_FUSION/GATING/FIND_UNASSOCIATED_CLUSTERS ==
  GatedMeasFlagArray : Inport
  Clusters : Inport  Port=2
  measCLUSTERS : Inport  Port=3
  Terminator : Terminator
  Terminator1 : Terminator
  UngatedCLUSTERS : Outport
  wires:
  measCLUSTERS/1 -> UngatedCLUSTERS/1
  GatedMeasFlagArray/1 -> Terminator/1
  Clusters/1 -> Terminator1/1

== system Fusion_Frame_Model_Architecture/SENSOR_FUSION_SYSTEM/OBJECT_TRACKER_SENSOR_FUSION/CAMERA_HOMOGENEOUS_FUSION/GATING/GET_DATA ==
  TRACKS : Inport
  Bus Selector : BusSelector  OutputSignals=nValidTracks,TrackParam
  nTracksPred : Outport
  TrackParam : Outport  Port=2
  wires:
  TRACKS/1 -> Bus Selector/1
  Bus Selector/1 -> nTracksPred/1  "<nValidTracks>"
  Bus Selector/2 -> TrackParam/1  "<TrackParam>"

== system Fusion_Frame_Model_Architecture/SENSOR_FUSION_SYSTEM/OBJECT_TRACKER_SENSOR_FUSION/CAMERA_HOMOGENEOUS_FUSION/GATING/MEASUREMENT_TO_TRACK_GATING_AND_LOGLIKELIHOOD_COMPUTATION ==
  nTracks : Inport
  TrackParamPred : Inport  Port=2
  SnsrParam : Inport  Port=3
  Meas : Inport  Port=4
  For Iterator : ForIterator  ResetStates=reset  IterationSource=external
  GATE_MEASUREMENTS_AND_COMPUTE_LIKELIHOOD : Subsystem
  GET_DATA : Subsystem
  Terminator : Terminator
  Unit Delay : UnitDelay  InitialCondition=boolean(zeros(100, 1200))  SampleTime=-1
  Unit Delay1 : UnitDelay  InitialCondition=single(zeros(100, 1200))  SampleTime=-1
  nMeas : Outport
  GatedMeasFlagArray : Outport  Port=2
  GatedMeasLogLikelihood : Outport  Port=3
  wires:
  GATE_MEASUREMENTS_AND_COMPUTE_LIKELIHOOD/1(GatedMeasFlagArray) -> GatedMeasFlagArray/1, Unit Delay/1
  nTracks/1 -> For Iterator/1
  TrackParamPred/1 -> GET_DATA/2(TrackParamPred)
  GATE_MEASUREMENTS_AND_COMPUTE_LIKELIHOOD/2(LogLikelihoodArray) -> Unit Delay1/1, GatedMeasLogLikelihood/1
  GET_DATA/2(StateVector) -> GATE_MEASUREMENTS_AND_COMPUTE_LIKELIHOOD/4(TrackStateVector)
  GET_DATA/3(StateErrCov) -> GATE_MEASUREMENTS_AND_COMPUTE_LIKELIHOOD/5(TrackErrCov)
  For Iterator/1 -> GATE_MEASUREMENTS_AND_COMPUTE_LIKELIHOOD/6(TrackIdx), GET_DATA/3(TrackIdx)
  Meas/1 -> GATE_MEASUREMENTS_AND_COMPUTE_LIKELIHOOD/2(Meas), GET_DATA/1(Meas)
  GET_DATA/1(nMeas) -> [nMeas], GATE_MEASUREMENTS_AND_COMPUTE_LIKELIHOOD/3(nMeas)
  Unit Delay1/1 -> GATE_MEASUREMENTS_AND_COMPUTE_LIKELIHOOD/7(LogLikelihoodArrayIn)
  Unit Delay/1 -> GATE_MEASUREMENTS_AND_COMPUTE_LIKELIHOOD/1(GatedMeasFlagArrayIn)
  [nMeas] -> nMeas/1
  SnsrParam/1 -> Terminator/1

== system Fusion_Frame_Model_Architecture/SENSOR_FUSION_SYSTEM/OBJECT_TRACKER_SENSOR_FUSION/CAMERA_HOMOGENEOUS_FUSION/GATING/RESOLVE_GATING_AMBIGUITY ==
  nTracks : Inport
  nMeas : Inport  Port=2
  GatedMeasFlagArrayIn : Inport  Port=3
  GatedMeasLogLikelihoodIn : Inport  Port=4
  Terminator : Terminator
  Terminator1 : Terminator
  GatedMeasFlagArray : Outport
  GatedMeasLogLikelihood : Outport  Port=2
  wires:
  nTracks/1 -> Terminator/1
  GatedMeasLogLikelihoodIn/1 -> GatedMeasLogLikelihood/1
  GatedMeasFlagArrayIn/1 -> GatedMeasFlagArray/1
  nMeas/1 -> Terminator1/1

== system Fusion_Frame_Model_Architecture/SENSOR_FUSION_SYSTEM/OBJECT_TRACKER_SENSOR_FUSION/CAMERA_HOMOGENEOUS_FUSION/NEAREST_NEIGHBOUR_CLUSTERING_FOR_CAMERA_MEASUREMENT/GET_NUM_OF_MEAS ==
  CAM_MEAS_CTS : Inport
  Bus Selector : BusSelector  OutputSignals=ValidCumulativeMeasCount
  Selector : Selector  NumberOfDimensions=2  InputPortWidth=3  IndexOptions=Select all,Index vector (port)  Indices=[1 3],1  OutputSizes=1,1
  Width : Width
  nMeas : Outport
  wires:
  CAM_MEAS_CTS/1 -> Bus Selector/1
  Bus Selector/1 -> Width/1, Selector/1  "<ValidCumulativeMeasCount>"
  Selector/1 -> nMeas/1
  Width/1 -> Selector/2

== system Fusion_Frame_Model_Architecture/SENSOR_FUSION_SYSTEM/OBJECT_TRACKER_SENSOR_FUSION/CAMERA_HOMOGENEOUS_FUSION/NEAREST_NEIGHBOUR_CLUSTERING_FOR_CAMERA_MEASUREMENT/NN_MEASUREMENT_GROUPING_WITHIN_EPS ==
  nMeas : Inport
  Meas : Inport  Port=2
  COMPUTE_MEAN_IF_CLUSTER_FORMED : Subsystem
  For Iterator : ForIterator  ResetStates=reset  IterationSource=external
  For Iterator Subsystem : Subsystem  TreatAsAtomicUnit=on
  Subsystem1 : Subsystem
  Subsystem2 : Subsystem
  Subsystem3 : Subsystem
  CAMERA_CLUSTERS : Outport
  wires:
  nMeas/1 -> For Iterator/1
  For Iterator/1 -> For Iterator Subsystem/1(idx_i)
  Meas/1 -> [meas], For Iterator Subsystem/2(measArray)
  For Iterator Subsystem/2(CLSTR_DATA_out) -> COMPUTE_MEAN_IF_CLUSTER_FORMED/2(CLSTR_DATA), Subsystem3/5(CLSTR_DATA)
  Subsystem1/2(Upd) -> COMPUTE_MEAN_IF_CLUSTER_FORMED/Enable
  Subsystem1/1(NoUpd) -> Subsystem2/Enable
  COMPUTE_MEAN_IF_CLUSTER_FORMED/1(CLSTR_CNTR_UPD) -> Subsystem3/3(MeanUpd)
  Subsystem2/1(Mean) -> Subsystem3/1(MeanNoUpd)
  Subsystem2/2(Cov) -> Subsystem3/2(CovNoUpd)
  COMPUTE_MEAN_IF_CLUSTER_FORMED/2(CLSTR_COV_UPD) -> Subsystem3/4(CovUpd)
  Subsystem3/1(CLSTR_DATA_UPD) -> CAMERA_CLUSTERS/1, For Iterator Subsystem/3(CLSTR_DATA)
  [A] -> Subsystem3/6(Flag)
  For Iterator Subsystem/1(nPts) -> [A], Subsystem1/1(CLSTR_DATA)
  [meas] -> COMPUTE_MEAN_IF_CLUSTER_FORMED/1(meas)

== system Fusion_Frame_Model_Architecture/SENSOR_FUSION_SYSTEM/OBJECT_TRACKER_SENSOR_FUSION/CAMERA_HOMOGENEOUS_FUSION/STATE_PREDICTION/GET_DATA ==
  TRACKS : Inport
  Bus Selector : BusSelector  OutputSignals=nValidTracks,TrackParam
  nTracksPrev : Outport
  TrackParam : Outport  Port=2
  wires:
  TRACKS/1 -> Bus Selector/1
  Bus Selector/1 -> nTracksPrev/1  "<nValidTracks>"
  Bus Selector/2 -> TrackParam/1  "<TrackParam>"

== system Fusion_Frame_Model_Architecture/SENSOR_FUSION_SYSTEM/OBJECT_TRACKER_SENSOR_FUSION/CAMERA_HOMOGENEOUS_FUSION/STATE_PREDICTION/SET_DATA ==
  TRACKS_in : Inport
  TrackParam : Inport  Port=2
  Bus Creator : BusCreator  Inputs=6  OutDataTypeStr=Bus: TRACK_ESTIMATES_BUS  NonVirtualBus=on
      settings: InheritFromInputs=off
  Bus Selector : BusSelector  OutputSignals=nValidTracks,TrackParam,TrackIDList,IsTrackIDused,FirstAvailableIDindex,LastAvailableIDindex
  Terminator : Terminator
  TRACKS : Outport
  wires:
  Bus Creator/1 -> TRACKS/1
  Bus Selector/3 -> Bus Creator/3  "<TrackIDList>"
  Bus Selector/2 -> Terminator/1  "<TrackParam>"
  Bus Selector/6 -> Bus Creator/6  "<LastAvailableIDindex>"
  Bus Selector/5 -> Bus Creator/5  "<FirstAvailableIDindex>"
  Bus Selector/1 -> Bus Creator/1  "<nValidTracks>"
  TRACKS_in/1 -> Bus Selector/1
  TrackParam/1 -> Bus Creator/2  "TrackParam"
  Bus Selector/4 -> Bus Creator/4  "<IsTrackIDused>"

== system Fusion_Frame_Model_Architecture/SENSOR_FUSION_SYSTEM/OBJECT_TRACKER_SENSOR_FUSION/CAMERA_HOMOGENEOUS_FUSION/STATE_PREDICTION/TRACK_STATE_PREDICTION ==
  nTracks : Inport
  TrackParamPred : Inport  Port=2
  For Iterator : ForIterator  ResetStates=reset  IterationSource=external
  GET_DATA : Subsystem
  SET_DATA : Subsystem
  StatePredictionLinearModels : Subsystem
  StatePredBus : Outport
  wires:
  nTracks/1 -> For Iterator/1
  TrackParamPred/1 -> SET_DATA/4(StateParamArray), GET_DATA/1(TrackParamPred)
  GET_DATA/1(StateVector) -> StatePredictionLinearModels/1(StateVectorCA)
  GET_DATA/2(StateErrCov) -> StatePredictionLinearModels/2(PrevStateErrorCov)
  StatePredictionLinearModels/1(StatePred) -> SET_DATA/1(StatePred)
  StatePredictionLinearModels/2(PriorStateErrorCov) -> SET_DATA/2(PredStateErrCov)
  SET_DATA/1(StateParam) -> StatePredBus/1
  For Iterator/1 -> SET_DATA/3(objIdx), GET_DATA/2(TrackIdx)

== system Fusion_Frame_Model_Architecture/SENSOR_FUSION_SYSTEM/OBJECT_TRACKER_SENSOR_FUSION/RADAR_HOMOGENEOUS_FUSION/GATING/FIND_UNASSOCIATED_CLUSTERS ==
  GatedMeasFlagArray : Inport
  Clusters : Inport  Port=2
  measCLUSTERS : Inport  Port=3
  Terminator : Terminator
  Terminator1 : Terminator
  UngatedCLUSTERS : Outport
  wires:
  measCLUSTERS/1 -> UngatedCLUSTERS/1
  GatedMeasFlagArray/1 -> Terminator/1
  Clusters/1 -> Terminator1/1

== system Fusion_Frame_Model_Architecture/SENSOR_FUSION_SYSTEM/OBJECT_TRACKER_SENSOR_FUSION/RADAR_HOMOGENEOUS_FUSION/GATING/GET_DATA ==
  TRACKS : Inport
  Bus Selector : BusSelector  OutputSignals=nValidTracks,TrackParam
  nTracksPred : Outport
  TrackParam : Outport  Port=2
  wires:
  TRACKS/1 -> Bus Selector/1
  Bus Selector/1 -> nTracksPred/1  "<nValidTracks>"
  Bus Selector/2 -> TrackParam/1  "<TrackParam>"

== system Fusion_Frame_Model_Architecture/SENSOR_FUSION_SYSTEM/OBJECT_TRACKER_SENSOR_FUSION/RADAR_HOMOGENEOUS_FUSION/GATING/MEASUREMENT_TO_TRACK_GATING_AND_LOGLIKELIHOOD_COMPUTATION ==
  nTracks : Inport
  TrackParamPred : Inport  Port=2
  SnsrParam : Inport  Port=3
  Meas : Inport  Port=4
  For Iterator : ForIterator  ResetStates=reset  IterationSource=external
  GATE_MEASUREMENTS_AND_COMPUTE_LIKELIHOOD : Subsystem
  GET_DATA : Subsystem
  Unit Delay : UnitDelay  InitialCondition=boolean(zeros(100, 1200))  SampleTime=-1
  Unit Delay1 : UnitDelay  InitialCondition=single(zeros(100, 1200))  SampleTime=-1
  nMeas : Outport
  GatedMeasFlagArray : Outport  Port=2
  GatedMeasLogLikelihood : Outport  Port=3
  wires:
  GATE_MEASUREMENTS_AND_COMPUTE_LIKELIHOOD/1(GatedMeasFlagArray) -> Unit Delay/1, GatedMeasFlagArray/1
  nTracks/1 -> For Iterator/1
  TrackParamPred/1 -> GET_DATA/2(TrackParamPred)
  GATE_MEASUREMENTS_AND_COMPUTE_LIKELIHOOD/2(LogLikelihoodArray1) -> Unit Delay1/1, GatedMeasLogLikelihood/1
  GET_DATA/2(StateVector) -> GATE_MEASUREMENTS_AND_COMPUTE_LIKELIHOOD/4(TrackStateVector)
  GET_DATA/3(StateErrCov) -> GATE_MEASUREMENTS_AND_COMPUTE_LIKELIHOOD/5(TrackErrCov)
  For Iterator/1 -> GATE_MEASUREMENTS_AND_COMPUTE_LIKELIHOOD/6(TrackIdx), GET_DATA/3(TrackIdx)
  Meas/1 -> GATE_MEASUREMENTS_AND_COMPUTE_LIKELIHOOD/2(Meas), GET_DATA/1(Meas)
  GET_DATA/1(nMeas) -> [nMeas], GATE_MEASUREMENTS_AND_COMPUTE_LIKELIHOOD/3(nMeas)
  Unit Delay1/1 -> GATE_MEASUREMENTS_AND_COMPUTE_LIKELIHOOD/8(LogLikelihoodArrayIn)
  Unit Delay/1 -> GATE_MEASUREMENTS_AND_COMPUTE_LIKELIHOOD/1(GatedMeasFlagArrayIn)
  [nMeas] -> nMeas/1
  SnsrParam/1 -> GATE_MEASUREMENTS_AND_COMPUTE_LIKELIHOOD/7(SnsrParam)

== system Fusion_Frame_Model_Architecture/SENSOR_FUSION_SYSTEM/OBJECT_TRACKER_SENSOR_FUSION/RADAR_HOMOGENEOUS_FUSION/GATING/RESOLVE_GATING_AMBIGUITY ==
  nTracks : Inport
  nMeas : Inport  Port=2
  GatedMeasFlagArrayIn : Inport  Port=3
  GatedMeasLogLikelihoodIn : Inport  Port=4
  Terminator : Terminator
  Terminator1 : Terminator
  GatedMeasFlagArray : Outport
  GatedMeasLogLikelihood : Outport  Port=2
  wires:
  nMeas/1 -> Terminator/1
  nTracks/1 -> Terminator1/1
  GatedMeasFlagArrayIn/1 -> GatedMeasFlagArray/1
  GatedMeasLogLikelihoodIn/1 -> GatedMeasLogLikelihood/1

== system Fusion_Frame_Model_Architecture/SENSOR_FUSION_SYSTEM/OBJECT_TRACKER_SENSOR_FUSION/RADAR_HOMOGENEOUS_FUSION/SEGREGATE_CLUSTER/Spatially_Alligned_Snsr_Meas_Plots ==
  RAD_MEAS : Inport
  Bus Selector : BusSelector  OutputSignals=MeasArray,ValidCumulativeMeasCount
  RadarMeasCTS : Scope
  Selector : Selector  NumberOfDimensions=2  InputPortWidth=3  IndexOptions=Select all,Index vector (port)  Indices=[1 3],1  OutputSizes=1,1
  Selector1 : Selector  NumberOfDimensions=2  InputPortWidth=3  IndexOptions=Index vector (dialog),Index vector (dialog)  Indices=1,1:30  OutputSizes=1,1
  Width : Width
  nRadarMeasurements : Scope
  wires:
  Bus Selector/1 -> Selector1/1  "<MeasArray>"
  Bus Selector/2 -> Selector/1, Width/1  "<ValidCumulativeMeasCount>"
  Width/1 -> Selector/2
  Selector1/1 -> RadarMeasCTS/1
  RAD_MEAS/1 -> Bus Selector/1
  Selector/1 -> nRadarMeasurements/1

== system Fusion_Frame_Model_Architecture/SENSOR_FUSION_SYSTEM/OBJECT_TRACKER_SENSOR_FUSION/RADAR_HOMOGENEOUS_FUSION/SIMPLYFIED_DBSCAN_FOR_RADAR_MEASUREMENT_GROUPING/DBSCAN_MEASUREMENT_GROUPING ==
  nMeas : Inport
  Meas : Inport  Port=2
  CHECK_IF_CLUSTER_FORMED : Subsystem
  COMPUTE_MEAN_IF_CLUSTER_FORMED : Subsystem
  FORM_CLUSTER : Subsystem  TreatAsAtomicUnit=on
  For Iterator : ForIterator  ResetStates=reset  IterationSource=external
  IF_CLUSTER_NOT_FORMED : Subsystem
  MERGE_SIGNALS : Subsystem
  RADAR_CLUSTERS : Outport
  wires:
  nMeas/1 -> For Iterator/1
  For Iterator/1 -> FORM_CLUSTER/1(idx_i)
  Meas/1 -> [meas], FORM_CLUSTER/2(measArray)
  FORM_CLUSTER/2(isMeasVisited) -> COMPUTE_MEAN_IF_CLUSTER_FORMED/1(CLSTR_DATA), MERGE_SIGNALS/5(CLSTR_DATA)
  CHECK_IF_CLUSTER_FORMED/2(Upd) -> COMPUTE_MEAN_IF_CLUSTER_FORMED/Enable
  CHECK_IF_CLUSTER_FORMED/1(NoUpd) -> IF_CLUSTER_NOT_FORMED/Enable
  COMPUTE_MEAN_IF_CLUSTER_FORMED/1(CLSTR_CNTR_UPD) -> MERGE_SIGNALS/3(MeanUpd)
  IF_CLUSTER_NOT_FORMED/1(Mean) -> MERGE_SIGNALS/1(MeanNoUpd)
  IF_CLUSTER_NOT_FORMED/2(Cov) -> MERGE_SIGNALS/2(CovNoUpd)
  COMPUTE_MEAN_IF_CLUSTER_FORMED/2(CLSTR_COV_UPD) -> MERGE_SIGNALS/4(CovUpd)
  MERGE_SIGNALS/1(CLSTR_DATA_UPD) -> RADAR_CLUSTERS/1, FORM_CLUSTER/3(CLSTR_DATA)
  [meas] -> COMPUTE_MEAN_IF_CLUSTER_FORMED/2(meas)
  [A] -> MERGE_SIGNALS/6(Flag)
  FORM_CLUSTER/1(nPts) -> [A], CHECK_IF_CLUSTER_FORMED/1(nPts)

== system Fusion_Frame_Model_Architecture/SENSOR_FUSION_SYSTEM/OBJECT_TRACKER_SENSOR_FUSION/RADAR_HOMOGENEOUS_FUSION/SIMPLYFIED_DBSCAN_FOR_RADAR_MEASUREMENT_GROUPING/GET_NUM_OF_MEAS ==
  RAD_MEAS_CTS : Inport
  Bus Selector : BusSelector  OutputSignals=ValidCumulativeMeasCount
  Selector : Selector  NumberOfDimensions=2  InputPortWidth=3  IndexOptions=Select all,Index vector (port)  Indices=[1 3],1  OutputSizes=1,1
  Width : Width
  nMeas : Outport
  wires:
  RAD_MEAS_CTS/1 -> Bus Selector/1
  Bus Selector/1 -> Width/1, Selector/1  "<ValidCumulativeMeasCount>"
  Selector/1 -> nMeas/1
  Width/1 -> Selector/2

== system Fusion_Frame_Model_Architecture/SENSOR_FUSION_SYSTEM/OBJECT_TRACKER_SENSOR_FUSION/RADAR_HOMOGENEOUS_FUSION/STATE_PREDICTION/GET_DATA ==
  TRACKS : Inport
  Bus Selector : BusSelector  OutputSignals=nValidTracks,TrackParam
  nTracksPrev : Outport
  TrackParam : Outport  Port=2
  wires:
  TRACKS/1 -> Bus Selector/1
  Bus Selector/1 -> nTracksPrev/1  "<nValidTracks>"
  Bus Selector/2 -> TrackParam/1  "<TrackParam>"

== system Fusion_Frame_Model_Architecture/SENSOR_FUSION_SYSTEM/OBJECT_TRACKER_SENSOR_FUSION/RADAR_HOMOGENEOUS_FUSION/STATE_PREDICTION/SET_DATA ==
  TRACKS_in : Inport
  TrackParam : Inport  Port=2
  Bus Creator : BusCreator  Inputs=6  OutDataTypeStr=Bus: TRACK_ESTIMATES_BUS  NonVirtualBus=on
      settings: InheritFromInputs=off
  Bus Selector : BusSelector  OutputSignals=nValidTracks,TrackParam,TrackIDList,IsTrackIDused,FirstAvailableIDindex,LastAvailableIDindex
  Terminator : Terminator
  TRACKS : Outport
  wires:
  Bus Creator/1 -> TRACKS/1
  Bus Selector/3 -> Bus Creator/3  "<TrackIDList>"
  Bus Selector/2 -> Terminator/1  "<TrackParam>"
  Bus Selector/6 -> Bus Creator/6  "<LastAvailableIDindex>"
  Bus Selector/5 -> Bus Creator/5  "<FirstAvailableIDindex>"
  Bus Selector/1 -> Bus Creator/1  "<nValidTracks>"
  TRACKS_in/1 -> Bus Selector/1
  TrackParam/1 -> Bus Creator/2  "TrackParam"
  Bus Selector/4 -> Bus Creator/4  "<IsTrackIDused>"

== system Fusion_Frame_Model_Architecture/SENSOR_FUSION_SYSTEM/OBJECT_TRACKER_SENSOR_FUSION/RADAR_HOMOGENEOUS_FUSION/STATE_PREDICTION/TRACK_STATE_PREDICTION ==
  nTracks : Inport
  TrackParamPred : Inport  Port=2
  For Iterator : ForIterator  ResetStates=reset  IterationSource=external
  GET_DATA : Subsystem
  SET_DATA : Subsystem
  StatePredictionLinearModels : Subsystem
  StatePredBus : Outport
  wires:
  nTracks/1 -> For Iterator/1
  TrackParamPred/1 -> SET_DATA/4(StateParamArray), GET_DATA/1(TrackParamPred)
  GET_DATA/1(StateVector) -> StatePredictionLinearModels/1(StateVectorCA)
  GET_DATA/2(StateErrCov) -> StatePredictionLinearModels/2(PrevStateErrorCov)
  StatePredictionLinearModels/1(StatePred) -> SET_DATA/1(StatePred)
  StatePredictionLinearModels/2(PriorStateErrorCov) -> SET_DATA/2(PredStateErrCov)
  SET_DATA/1(StateParam) -> StatePredBus/1
  For Iterator/1 -> SET_DATA/3(objIdx), GET_DATA/2(TrackIdx)

== system Fusion_Frame_Model_Architecture/SENSOR_FUSION_SYSTEM/OBJECT_TRACKER_SENSOR_FUSION/SENSOR_LAYOUT_AND_CHRACTERIZATION/PRE_COMPUTE_SENSOR_FOV_GRID/COMPUTE_CAMERA_SNSR_GRID ==
  GridIDVector : Inport
  GridParam : Inport  Port=2
  SnsrParam : Inport  Port=3
  ComputeCoverageANDConfidence : Subsystem  TreatAsAtomicUnit=on
  GET_SENSOR_PARAMETERS : Subsystem
  SENSOR_LOOP : ForIterator  ResetStates=reset  IterationLimit=nCameras  IterationVariableDataType=int8
  Unit Delay : UnitDelay  InitialCondition=RegionConfidenceCAM  SampleTime=-1
  Unit Delay1 : UnitDelay  InitialCondition=FOVOverlapCAM  SampleTime=-1
  Width : Width
  RegionConfidence : Outport
  FOVOverlap : Outport  Port=2
  wires:
  GridIDVector/1 -> ComputeCoverageANDConfidence/3(GridIDVector), Width/1
  Width/1 -> ComputeCoverageANDConfidence/2(nGridCells)
  SENSOR_LOOP/1 -> ComputeCoverageANDConfidence/5(SensorID), GET_SENSOR_PARAMETERS/1(SensorID)
  SnsrParam/1 -> GET_SENSOR_PARAMETERS/2(SensorParam)
  GET_SENSOR_PARAMETERS/1(extrinsic) -> ComputeCoverageANDConfidence/6(SensorExtrinsic)
  GET_SENSOR_PARAMETERS/2(intrinsic) -> ComputeCoverageANDConfidence/7(SensorIntrinsic)
  GridParam/1 -> ComputeCoverageANDConfidence/4(GridParam)
  ComputeCoverageANDConfidence/1(RegionConfidence) -> Unit Delay/1, RegionConfidence/1
  ComputeCoverageANDConfidence/2(FOVOverlap) -> Unit Delay1/1, FOVOverlap/1
  Unit Delay/1 -> ComputeCoverageANDConfidence/1(RegionConfidenceArray)
  Unit Delay1/1 -> ComputeCoverageANDConfidence/8(FOVOverlapArray)

== system Fusion_Frame_Model_Architecture/SENSOR_FUSION_SYSTEM/OBJECT_TRACKER_SENSOR_FUSION/SENSOR_LAYOUT_AND_CHRACTERIZATION/PRE_COMPUTE_SENSOR_FOV_GRID/COMPUTE_GRID_DIMENSION ==
  note: Set_Grid_Parameters
  note: Compute_number_of_grid_cells
  note: Compute_number_of_logitudinal_Grid_Cells
  note: Compute_number_of_lateral_Grid_Cells
  Bus Creator1 : BusCreator  Inputs=3  OutDataTypeStr=Bus: GRID_PARAM  NonVirtualBus=on
      settings: InheritFromInputs=off
  Bus Creator2 : BusCreator  Inputs=4  OutDataTypeStr=Bus: yGridParameters  NonVirtualBus=on
      settings: InheritFromInputs=off
  Bus Creator3 : BusCreator  Inputs=4  OutDataTypeStr=Bus: xGridParameters  NonVirtualBus=on
      settings: InheritFromInputs=off
  Constant1 : Constant  Value=single(1)
  Constant3 : Constant  Value=single(1)
  Data Type Conversion : DataTypeConversion  OutDataTypeStr=int32
  Data Type Conversion1 : DataTypeConversion  OutDataTypeStr=int32
  Data Type Conversion3 : DataTypeConversion  OutDataTypeStr=int32
  Divide : Product  Inputs=*/
  Divide1 : Product  Inputs=/*
  Divide2 : Product  Inputs=*/
  Divide3 : Product  Inputs=/*
  Floor{,1..3} (4 alike) : Rounding
  Gain : Gain  Gain=single(-1)
  Gain1 : Gain  Gain=single(-1)
  GridFrontLimit : Constant  Value=xFront
  GridLeftLimit : Constant  Value=yLeft
  GridRearLimit : Constant  Value=xRear
  GridResLat : Constant  Value=yRes
  GridResLong : Constant  Value=xRes
  GridRightLimit : Constant  Value=yRight
  Minus : Sum  Inputs=+-+
  Minus1 : Sum  Inputs=+-+
  Multiply : Product
  Saturation : Saturate  UpperLimit=10  LowerLimit=0.5
  Saturation1 : Saturate  UpperLimit=10  LowerLimit=0.5
  Cx : Outport
  Cy : Outport  Port=2
  GridParam : Outport  Port=3
  wires:
  GridResLong/1 -> Saturation/1
  Saturation/1 -> [xRes], Divide1/1, Divide/2
  GridFrontLimit/1 -> [xFront], Divide/1
  Divide/1 -> Floor/1
  GridRearLimit/1 -> Gain/1
  Gain/1 -> [xRear], Divide1/2
  Divide1/1 -> Floor1/1
  Floor/1 -> Minus/1
  Floor1/1 -> Minus/2
  Constant1/1 -> Minus/3
  Divide2/1 -> Floor2/1
  GridRightLimit/1 -> [yRight], Divide2/1
  GridResLat/1 -> Saturation1/1
  Constant3/1 -> Minus1/3
  Saturation1/1 -> [yRes], Divide3/1, Divide2/2
  GridLeftLimit/1 -> Gain1/1
  Gain1/1 -> [yLeft], Divide3/2
  Floor2/1 -> Minus1/1
  Divide3/1 -> Floor3/1
  Floor3/1 -> Minus1/2
  Minus/1 -> Multiply/1, Data Type Conversion/1
  Minus1/1 -> Multiply/2, Data Type Conversion3/1
  Data Type Conversion/1 -> [nGridCellsLong]
  Multiply/1 -> Data Type Conversion1/1
  Data Type Conversion1/1 -> [nGridCells]
  [nGridCells] -> Bus Creator1/1  "nGridCells"
  [nGridCellsLat] -> Cy/1, Bus Creator2/1  "nGridCellsLat"
  [yRes] -> Bus Creator2/2  "yRes"
  [yRight] -> Bus Creator2/3  "yRight"
  [yLeft] -> Bus Creator2/4  "yLeft"
  Bus Creator2/1 -> Bus Creator1/3  "yGridParameters"
  Data Type Conversion3/1 -> [nGridCellsLat]
  [nGridCellsLong] -> Cx/1, Bus Creator3/1  "nGridCellsLong"
  [xRear] -> Bus Creator3/4  "xRear"
  Bus Creator3/1 -> Bus Creator1/2  "xGridParameters"
  [xRes] -> Bus Creator3/2  "xRes"
  [xFront] -> Bus Creator3/3  "xFront"
  Bus Creator1/1 -> GridParam/1

== system Fusion_Frame_Model_Architecture/SENSOR_FUSION_SYSTEM/OBJECT_TRACKER_SENSOR_FUSION/SENSOR_LAYOUT_AND_CHRACTERIZATION/PRE_COMPUTE_SENSOR_FOV_GRID/COMPUTE_RADAR_SNSR_GRID ==
  SnsrParam : Inport
  GridParam : Inport  Port=2
  GridIDVector : Inport  Port=3
  ComputeCoverageANDConfidence : Subsystem  TreatAsAtomicUnit=on
  GET_SENSOR_PARAMETERS : Subsystem
  SENSOR_LOOP : ForIterator  ResetStates=reset  IterationLimit=nRadars  IterationVariableDataType=int8
  Unit Delay : UnitDelay  InitialCondition=RegionConfidenceRAD  SampleTime=-1
  Unit Delay1 : UnitDelay  InitialCondition=FOVOverlapRAD  SampleTime=-1
  Width : Width
  RegionConfidence : Outport
  FOVOverlap : Outport  Port=2
  wires:
  GridIDVector/1 -> ComputeCoverageANDConfidence/3(GridIDVector), Width/1
  Width/1 -> ComputeCoverageANDConfidence/2(nGridCells)
  SENSOR_LOOP/1 -> ComputeCoverageANDConfidence/5(SensorID), GET_SENSOR_PARAMETERS/1(SensorID)
  SnsrParam/1 -> GET_SENSOR_PARAMETERS/2(SensorParam)
  GET_SENSOR_PARAMETERS/1(extrinsic) -> ComputeCoverageANDConfidence/6(SensorExtrinsic)
  GET_SENSOR_PARAMETERS/2(intrinsic) -> ComputeCoverageANDConfidence/7(SensorIntrinsic)
  GridParam/1 -> ComputeCoverageANDConfidence/4(GridParam)
  ComputeCoverageANDConfidence/1(RegionConfidence) -> Unit Delay/1, RegionConfidence/1
  ComputeCoverageANDConfidence/2(FOVOverlap) -> Unit Delay1/1, FOVOverlap/1
  Unit Delay/1 -> ComputeCoverageANDConfidence/1(RegionConfidenceArray)
  Unit Delay1/1 -> ComputeCoverageANDConfidence/8(FOVOverlapArray)

== system Fusion_Frame_Model_Architecture/SENSOR_FUSION_SYSTEM/OBJECT_TRACKER_SENSOR_FUSION/SENSOR_LAYOUT_AND_CHRACTERIZATION/PRE_COMPUTE_SENSOR_FOV_GRID/CREATE_GRID ==
  Cx : Inport
  Cy : Inport  Port=2
  GridParam : Inport  Port=3
  For Iterator : ForIterator  ResetStates=reset  IterationSource=external
  For Iterator Subsystem : Subsystem  TreatAsAtomicUnit=on
  Unit Delay : UnitDelay  InitialCondition=GridCellIDs  SampleTime=-1
  CellIDVectorUpd : Outport
  wires:
  For Iterator/1 -> For Iterator Subsystem/1(xIndex)
  GridParam/1 -> For Iterator Subsystem/3(GridParam)
  Cx/1 -> For Iterator/1
  Cy/1 -> For Iterator Subsystem/2(Cy)
  For Iterator Subsystem/1(CellIDVectorUpd) -> Unit Delay/1, CellIDVectorUpd/1
  Unit Delay/1 -> For Iterator Subsystem/4(CellIDArray)
